simulink model "CONTROL_SYSTEM_V2"  (R2024a)
settings: Solver=ode1  StartTime=0.0  StopTime=inf  FixedStep=0.01  RelTol=1e-5
values from neighbouring files (symbols this model uses):
  B_aet = 0.1503    [ESP32_CONTROL_SYSTEM_VAR_V2.m]
  Beta1 = 3*Omega_o    (= 150)    [ESP32_CONTROL_SYSTEM_VAR_V2.m]
  Beta2 = 3*(Omega_o^2)    (= 7500)    [ESP32_CONTROL_SYSTEM_VAR_V2.m]
  Beta3 = (Omega_o^3)    (= 125000)    [ESP32_CONTROL_SYSTEM_VAR_V2.m]
  Desire_Max = 255    [ESP32_CONTROL_SYSTEM_VAR_V2.m]
  Desire_Min = 0    [ESP32_CONTROL_SYSTEM_VAR_V2.m]
  Direction_Pin = 1    [ESP32_CONTROL_SYSTEM_VAR_V2.m]
  EN_Pin = 0    [ESP32_CONTROL_SYSTEM_VAR_V2.m]
  F_so = 0.089    [ESP32_CONTROL_SYSTEM_VAR_V2.m]
  J_aet = 0.0035    [ESP32_CONTROL_SYSTEM_VAR_V2.m]
  K_sp = 0.038586    [ESP32_CONTROL_SYSTEM_VAR_V2.m]
  Kd = 0.42    [ESP32_CONTROL_SYSTEM_VAR_V2.m]
  Ki = 2    [ESP32_CONTROL_SYSTEM_VAR_V2.m]
  Kp = 3    [ESP32_CONTROL_SYSTEM_VAR_V2.m]
  omga_c = 2    [ESP32_CONTROL_SYSTEM_VAR_V2.m]
  roa = 0.24    [ESP32_CONTROL_SYSTEM_VAR_V2.m]
  theta_o = 12    [ESP32_CONTROL_SYSTEM_VAR_V2.m]
  Toa_ho = 0.3193    [ESP32_CONTROL_SYSTEM_VAR_V2.m]
undefined symbols (not defined in the file or in its folder): Kn, sigbuilder_block
libraries: arduinolib x29, simulink_extras x12, slpidlib x3, spsOnDelayLib x2, simulink x2, slctrl_autotuning x2
(part 3 of 3)

== system CONTROL_SYSTEM_V2/Subsystem2/TB_Feedbakc Range Conversion1 ==
  Control Output : Inport
  TB_maxVal : Inport  Port=2
  TB_minVal : Inport  Port=3
  Add2 : Sum  Inputs=+-
  Add3 : Sum  Inputs=+-
  Constant : Constant
  Constant1 : Constant  Value=0
  Display1 : Display
  Display3 : Display
  Divide1 : Product  Inputs=*/
  Product1 : Product
  Subtract : Sum  Inputs=+-
  Sum : Sum
  0 - 100 Output1 : Outport
  wires:
  Subtract/1 -> Product1/2
  Sum/1 -> 0 - 100 Output1/1
  Product1/1 -> Sum/2
  Constant/1 -> Add2/1
  Add2/1 -> Display1/1, Divide1/1
  Constant1/1 -> Add2/2, Sum/1
  TB_maxVal/1 -> Add3/1
  Add3/1 -> Divide1/2, Display3/1
  Divide1/1 -> Product1/1
  Control Output/1 -> Subtract/1
  TB_minVal/1 -> Subtract/2, Add3/2

== system CONTROL_SYSTEM_V2/Subsystem6/FP_Input Range Conversion2 ==
  Control Output : Inport
  FP_maxVal : Inport  Port=2
  FP_minVal : Inport  Port=3
  Add2 : Sum  Inputs=+-
  Add3 : Sum  Inputs=+-
  Desire Max Value : Constant  Value=Desire_Max
  Desire Min Value : Constant  Value=Desire_Min
  Display1 : Display
  Display3 : Display
  Divide1 : Product  Inputs=*/
  Product1 : Product
  Subtract : Sum  Inputs=+-
  Sum : Sum
  0 - 255 Output : Outport
  wires:
  Control Output/1 -> Subtract/1
  FP_maxVal/1 -> Add3/1
  Add3/1 -> Divide1/2, Display3/1
  FP_minVal/1 -> Subtract/2, Add3/2
  Desire Min Value/1 -> Add2/2, Sum/1
  Subtract/1 -> Product1/2
  Desire Max Value/1 -> Add2/1
  Add2/1 -> Display1/1, Divide1/1
  Divide1/1 -> Product1/1
  Product1/1 -> Sum/2
  Sum/1 -> 0 - 255 Output/1

== system CONTROL_SYSTEM_V2/Subsystem6/H-Bridge Setting2 ==
  1 - 100 : Inport
  Digital Output : arduinolib/Digital Output  pinNumber=0  Direction=output  blockPlatform=arduino
  Digital Output1 : arduinolib/Digital Output  pinNumber=16  Direction=output  blockPlatform=arduino
  Direction Pin : Constant  Value=Direction_Pin
  Display3 : Display
  Display4 : Display
  Enable Pin : Constant  Value=EN_Pin
  PWM : arduinolib/PWM  pinNumber=4  frequencyType=Specify  desiredFrequency=19000  achievableFrequency=19000
  wires:
  Enable Pin/1 -> Display4/1, Digital Output/1
  1 - 100/1 -> PWM/1
  Direction Pin/1 -> Display3/1, Digital Output1/1

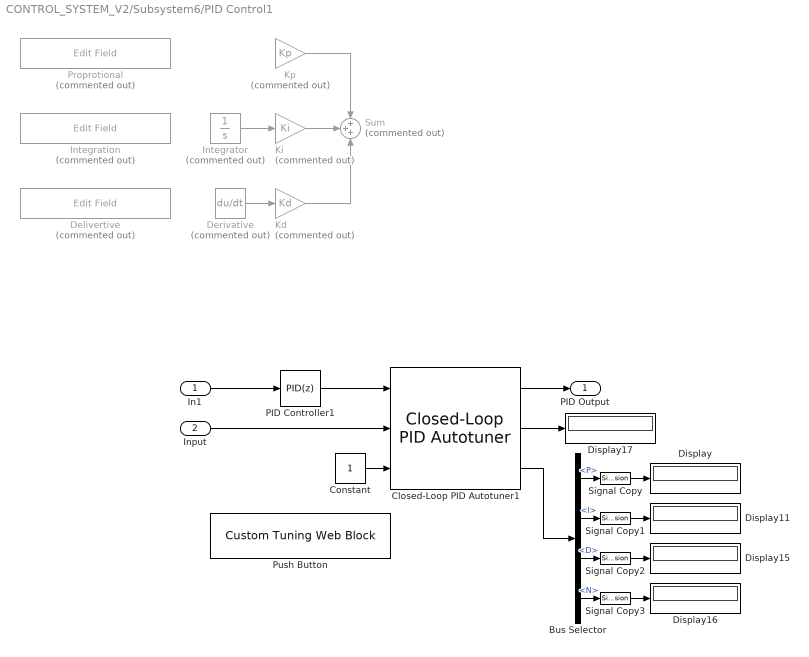
== system CONTROL_SYSTEM_V2/Subsystem6/PID Control1 ==
  In1 : Inport
  Input : Inport  Port=2
  Bus Selector : BusSelector  OutputSignals=P,I,D,N
  Closed-Loop PID Autotuner1 : slctrl_autotuning/Closed-Loop PID Autotuner  PIDType=PI  PIDForm=Parallel  TimeDomain=discrete-time  DiscreteTs=0.1  TuningTs=0.2  UseTuningTs=off  IntegratorFormula=Forward Euler  FilterFormula=Forward Euler  ContinuousTs=0.02  Bandwidth=1  UseExternalWC=off  TargetPM=60  UseExternalPM=off  UseExternalAchievedPM=off  ExperimentMode=Superposition  PlantType=Stable  PlantSign=Positive  AmpSine=1  UseExternalAmpSine=off  UseExternalFRD=off  UseExternalU0=off  UseCompanion=off  NotDeployTuningModule=off  UsePLCCoder=off  OutputMode=control action + perturbation  BlockDataType=double  UseConnectedPID=on  blockpath=[]  tunedP=0  tunedI=0  tunedD=0  tunedN=100  tunedPM=0  EstimationWindowSize=3  UseExternalTuningParams=off  SingleMultiRateVariant=SingleSamplingRate  NumEstimationPeriods=4  NumSettlingPeriods=2  NumOfPRBSPeriod=1  PRBSSignalOrder=12  ExperimentModeVariant=VariantSuperimposed  OutputChoice=VariantCandD
      settings: LibrarySourceBlock=slctrlblks/Autotuning/Closed-Loop PID Autotuner
  Constant : Constant
  Delivertive : EditField  Commented=on  LabelPosition=Hide  ShowInitialText=on  Alignment=Center
  Derivative : Derivative  Commented=on
  Display{,11,15..17} (5 alike) : Display
  Integration : EditField  Commented=on  LabelPosition=Hide  ShowInitialText=on  Alignment=Center
  Integrator : Integrator  Commented=on
  Kd : Gain  Commented=on  Gain=Kd
  Ki : Gain  Commented=on  Gain=Ki
  Kp : Gain  Commented=on  Gain=Kp
  PID Controller1 : slpidlib/PID Controller  Controller=PID  Form=Parallel  TimeDomain=Discrete-time  UseExternalTs=off  SampleTime=-1  IntegratorMethod=Forward Euler  FilterMethod=Forward Euler  ControllerParametersSource=internal  P=1  I=1  UseKiTs=off  D=0  UseExternalDerivativeSource=off  N=100  UseFilter=on  TunerSelectOption=Transfer Function Based (PID Tuner App)  InitialConditionSource=internal  InitialConditionForIntegrator=0  InitialConditionForFilter=0  DifferentiatorICPrevScaledInput=0  ExternalReset=none  TrackingMode=off  Kt=1  LimitOutput=off  SatLimitsSource=internal  UpperSaturationLimit=inf  LowerSaturationLimit=-inf  LinearizeAsGain=on  AntiWindupMode=none  Kb=1  LimitIntegrator=off  UpperIntegratorSaturationLimit=inf  LowerIntegratorSaturationLimit=-inf  POutMin=[]  POutMax=[]  IOutMin=[]  IOutMax=[]  DOutMin=[]  DOutMax=[]  NOutMin=[]  NOutMax=[]  SumOutMin=[]  SumOutMax=[]  SaturationOutMin=[]  SaturationOutMax=[]  PParamMin=[]  PParamMax=[]  IParamMin=[]  IParamMax=[]  DParamMin=[]  DParamMax=[]  NParamMin=[]  NParamMax=[]  KbParamMin=[]  KbParamMax=[]  KtParamMin=[]  KtParamMax=[]  KbOutMin=[]  KbOutMax=[]  KtOutMin=[]  KtOutMax=[]  IntegratorOutMin=[]  IntegratorOutMax=[]  FilterOutMin=[]  FilterOutMax=[]  SumI1OutMin=[]  SumI1OutMax=[]  SumI2OutMin=[]  SumI2OutMax=[]  SumI3OutMin=[]  SumI3OutMax=[]  SumI4OutMin=[]  SumI4OutMax=[]  SumDOutMin=[]  SumDOutMax=[]  DifferentiatorOutMin=[]  DifferentiatorOutMax=[]  FilterDiffOutCoefMin=[]  FilterDiffOutCoefMax=[]  ReciprocalOutMin=[]  ReciprocalOutMax=[]  SumDenOutMin=[]  SumDenOutMax=[]  SumNumOutMin=[]  SumNumOutMax=[]  DivideOutMin=[]  DivideOutMax=[]  UdiffTsProdOutMin=[]  UdiffTsProdOutMax=[]  NTsProdOutMin=[]  NTsProdOutMax=[]  UintegralTsProdOutMin=[]  UintegralTsProdOutMax=[]  UngainTsProdOutMin=[]  UngainTsProdOutMax=[]  ClampingZeroOutDataTypeStr=Inherit: Inherit via back propagation  ClampingZeroOutMin=[]  ClampingZeroOutMax=[]  FilterDenConstantOutDataTypeStr=Inherit: Inherit via back propagation  FilterDenConstantOutMin=[]  FilterDenConstantOutMax=[]  PCopyOutDataTypeStr=Inherit: Inherit via back propagation  PCopyOutMin=[]  PCopyOutMax=[]  NCopyOutDataTypeStr=Inherit: Inherit via back propagation  NCopyOutMin=[]  NCopyOutMax=[]  IntegratorContinuousStateAttributes=''  IntegratorStateMustResolveToSignalObject=off  IntegratorRTWStateStorageClass=Auto  FilterContinuousStateAttributes=''  FilterStateMustResolveToSignalObject=off  FilterRTWStateStorageClass=Auto  ParallelPVariant=InternalParameters  IdealPVariant=Disabled  IVariant=InternalParameters  DVariant=InternalParameters  IntegratorVariant=Discrete  SatVariant=Disabled  AWVariant=Passthrough  PCopyVariant=Disabled  TRVariant=Disabled  FdbkBlocksVariant=Forward  IdealPFdbkVariant=Disabled  SatFdbkVariant=Disabled  DerivativeFilterVariant=ForwardEulerFilter  NVariant=InternalParameters  NCopyVariant=Disabled  FilterICVariant=InternalICsFilter  IntegratorICVariant=InternalICs  ExternalResetVariant=Disabled  TRSumVariant=Passthrough  SumFdbkVariant=Disabled  SumVariant=Sum_PID  TsampFilterVariant=InternalTs  TsampNgainVariant=Passthrough  TsampIntegralVariant=Disabled_SignalSpec  ExternalSaturationOutDataTypeStr=Inherit: Same as second input  DerivativeSourceVariant=ErrorSignal
  Proprotional : EditField  Commented=on  LabelPosition=Hide  ShowInitialText=on  Alignment=Center
  Push Button : CustomTuningWebBlock  LabelPosition=Hide  ShowInitialText=on  Configuration="{\"components\":[{\"name\":\"BackgroundImageComponent\",\"settings\":{\"image\":{\"size\":[0,0],\"src\":\"default\",\"srcOrientation\":\"horizontal\"},\"position\":[0,0,1,1],\"scaleMode\":\"0\"}},{\"name\":\"ButtonStateComponent\",\"settings\":{\"buttonType\":\"latch\",\"clickFcn\":\"\",\"image\":{\"size\":[180,45],\"srcOrientation\":\"Right\"},\"latched\":true,\"offValue\":0,\"onValue\":\"1\",\"position\":[0,0,1,1],\"pressDelay\":\"500\",\"pressFcn\":\"\",\"repeatInterval\":\"0\",\"states\":[{\"horizontalAlignment\":\"center\",\"image\":{\"position\":[0.04444444444444445,0.005555555555555536,0.9888888888888889,0.9111111111111111],\"size\":[0.9888888888888889,0.9111111111111111],\"src\":\"data:image\\/svg+xml;base64,PHN2ZyB4bWxucz0iaHR0cDovL3d3dy53My5vcmcvMjAwMC9zdmciIHhtbG5zOnhsaW5rPSJodHRwOi8vd3d3LnczLm9yZy8xOTk5L3hsaW5rIiB2aWV3Qm94PSIwIDAgMTc3LjI1IDQwLjg4Ij48ZGVmcz48c3R5bGU+LmNscy0xe2ZpbGw6dXJsKCNyYWRpYWwtZ3JhZGllbnQpO30uY2xzLTJ7ZmlsbDp1cmwoI2xpbmVhci1ncmFkaWVudCk7fS5jbHMtM3tmaWxsOnVybCgjbGluZWFyLWdyYWRpZW50LTIpO308L3N0eWxlPjxyYWRpYWxHcmFkaWVudCBpZD0icmFkaWFsLWdyYWRpZW50IiBjeD0iOTAuMDkiIGN5PSIyMi42NiIgcj0i ...(+2212 chars)\",\"srcOrientation\":\"Right\"},\"label\":{\"color\":[1,1,0.78,1],\"icon\":{\"size\":[0.1,0.375],\"src\":\"data:image\\/svg+xml;base64,PHN2ZyBpZD0iT2ZmIiB4bWxucz0iaHR0cDovL3d3dy53My5vcmcvMjAwMC9zdmciIHhtbG5zOnhsaW5rPSJodHRwOi8vd3d3LnczLm9yZy8xOTk5L3hsaW5rIiB2aWV3Qm94PSIwIDAgNTAgNTAiPjxkZWZzPjxzdHlsZT4uY2xzLTF7ZmlsbDojN2Y4MDgwO3N0cm9rZTojMjcyNjI2O3N0cm9rZS1taXRlcmxpbWl0OjEwO3N0cm9rZS13aWR0aDozcHg7fS5jbHMtMntmaWxsOnVybCgjbGluZWFyLWdyYWRpZW50KTt9PC9zdHlsZT48bGluZWFyR3JhZGllbnQgaWQ9ImxpbmVhci1ncmFkaWVudCIgeDE9IjI1IiB5MT0iOSIgeDI9IjI1IiB5Mj0iMzciIGdyYWRpZW50VW5pdHM9InVzZXJTcGFjZU9uVXNlIj48c3RvcCBvZmZzZXQ9IjAiIHN0b3AtY29sb3I9IiNmZmYiIHN0b3Atb3BhY2l0eT0iMC43NSIvPjxzdG9wIG9mZnNldD0iMSIgc3RvcC1jb2xvcj0iI2ZmZiIgc3RvcC1vcGFjaXR5PSIwIi8+PC9saW5lYXJHcmFkaWVudD48L2RlZnM+PGNpcmNsZSBjbGFzcz0iY2xzLTEiIGN4PSIyNSIgY3k9IjI1IiByPSIyMCIvPjxjaXJjbGUgY2xhc3M9ImNscy0yIiBjeD0iMjUiIGN5PSIyMyIgcj0iMTQiLz48L3N2Zz4=\",\"srcOrientation\":\"Right\"},\"iconPlacement\":\"left\",\"opacity\":1,\"show\":true,\"text\":{\"content\":\"Button\",\"font\":\"Helvetica\",\"fontSize\":14}},\"labelOffset\":[0,0],\"verticalAlignment\":\"middle\"},{\"horizontalAlignment\":\"center\",\"image\":{\"position\":[0.04444444444444445,0.005555555555555536,0.9888888888888889,0.9111111111111111],\"size\":[0.9888888888888889,0.9111111111111111],\"src\":\"data:image\\/svg+xml;base64,PHN2ZyB4bWxucz0iaHR0cDovL3d3dy53My5vcmcvMjAwMC9zdmciIHhtbG5zOnhsaW5rPSJodHRwOi8vd3d3LnczLm9yZy8xOTk5L3hsaW5rIiB2aWV3Qm94PSIwIDAgMTc3LjI1IDQwLjg4Ij48ZGVmcz48c3R5bGU+LmNscy0xe2ZpbGw6dXJsKCNyYWRpYWwtZ3JhZGllbnQpO30uY2xzLTJ7ZmlsbDp1cmwoI2xpbmVhci1ncmFkaWVudCk7fS5jbHMtM3tmaWxsOnVybCgjbGluZWFyLWdyYWRpZW50LTIpO308L3N0eWxlPjxyYWRpYWxHcmFkaWVudCBpZD0icmFkaWFsLWdyYWRpZW50IiBjeD0iOTAuMDkiIGN5PSIyMi42NiIgcj0i ...(+2216 chars)\",\"srcOrientation\":\"Right\"},\"label\":{\"color\":[1,1,0.78,1],\"icon\":{\"size\":[0.1,0.375],\"src\":\"data:image\\/svg+xml;base64,PHN2ZyB4bWxucz0iaHR0cDovL3d3dy53My5vcmcvMjAwMC9zdmciIHhtbG5zOnhsaW5rPSJodHRwOi8vd3d3LnczLm9yZy8xOTk5L3hsaW5rIiB2aWV3Qm94PSIwIDAgNTAgNTAiPjxkZWZzPjxzdHlsZT4uY2xzLTF7ZmlsbDojNmFiZDQ1O3N0cm9rZTojMjcyNjI2O3N0cm9rZS1taXRlcmxpbWl0OjEwO3N0cm9rZS13aWR0aDozcHg7fS5jbHMtMntmaWxsOnVybCgjbGluZWFyLWdyYWRpZW50KTt9PC9zdHlsZT48bGluZWFyR3JhZGllbnQgaWQ9ImxpbmVhci1ncmFkaWVudCIgeDE9IjI1IiB5MT0iOSIgeDI9IjI1IiB5Mj0iMzciIGdyYWRpZW50VW5pdHM9InVzZXJTcGFjZU9uVXNlIj48c3RvcCBvZmZzZXQ9IjAiIHN0b3AtY29sb3I9IiNmZmYiIHN0b3Atb3BhY2l0eT0iMC43NSIvPjxzdG9wIG9mZnNldD0iMSIgc3RvcC1jb2xvcj0iI2ZmZiIgc3RvcC1vcGFjaXR5PSIwIi8+PC9saW5lYXJHcmFkaWVudD48L2RlZnM+PGcgaWQ9Ik9uIj48Y2lyY2xlIGNsYXNzPSJjbHMtMSIgY3g9IjI1IiBjeT0iMjUiIHI9IjIwIi8+PGNpcmNsZSBjbGFzcz0iY2xzLTIiIGN4PSIyNSIgY3k9IjIzIiByPSIxNCIvPjwvZz48L3N2Zz4=\",\"srcOrientation\":\"Right\"},\"iconPlacement\":\"left\",\"opacity\":1,\"show\":true,\"text\":{\"content\":\"Button\",\"font\":\"Helvetica\",\"fontSize\":14}},\"labelOffset\":[0.025,0],\"verticalAlignment\":\"middle\"},{\"horizontalAlignment\":\"center\",\"image\":{\"position\":[0.04444444444444445,0.005555555555555536,0.9888888888888889,0.9111111111111111],\"size\":[0.9888888888888889,0.9111111111111111],\"src\":\"data:image\\/svg+xml;base64,PHN2ZyB4bWxucz0iaHR0cDovL3d3dy53My5vcmcvMjAwMC9zdmciIHhtbG5zOnhsaW5rPSJodHRwOi8vd3d3LnczLm9yZy8xOTk5L3hsaW5rIiB2aWV3Qm94PSIwIDAgMTc3LjI1IDQwLjg4Ij48ZGVmcz48c3R5bGU+LmNscy0xe2ZpbGw6dXJsKCNyYWRpYWwtZ3JhZGllbnQpO30uY2xzLTJ7ZmlsbDp1cmwoI2xpbmVhci1ncmFkaWVudCk7fS5jbHMtM3tmaWxsOnVybCgjbGluZWFyLWdyYWRpZW50LTIpO308L3N0eWxlPjxyYWRpYWxHcmFkaWVudCBpZD0icmFkaWFsLWdyYWRpZW50IiBjeD0iOTAuMDkiIGN5PSIyMi42NiIgcj0i ...(+2212 chars)\",\"srcOrientation\":\"Right\"},\"label\":{\"color\":[1,1,0.78,1],\"icon\":{\"size\":[0.1,0.375],\"src\":\"data:image\\/svg+xml;base64,PHN2ZyB4bWxucz0iaHR0cDovL3d3dy53My5vcmcvMjAwMC9zdmciIHhtbG5zOnhsaW5rPSJodHRwOi8vd3d3LnczLm9yZy8xOTk5L3hsaW5rIiB2aWV3Qm94PSIwIDAgNTAgNTAiPjxkZWZzPjxzdHlsZT4uY2xzLTF7ZmlsbDojNmFiZDQ1O3N0cm9rZTojMjcyNjI2O3N0cm9rZS1taXRlcmxpbWl0OjEwO3N0cm9rZS13aWR0aDozcHg7fS5jbHMtMntmaWxsOnVybCgjbGluZWFyLWdyYWRpZW50KTt9PC9zdHlsZT48bGluZWFyR3JhZGllbnQgaWQ9ImxpbmVhci1ncmFkaWVudCIgeDE9IjI1IiB5MT0iOSIgeDI9IjI1IiB5Mj0iMzciIGdyYWRpZW50VW5pdHM9InVzZXJTcGFjZU9uVXNlIj48c3RvcCBvZmZzZXQ9IjAiIHN0b3AtY29sb3I9IiNmZmYiIHN0b3Atb3BhY2l0eT0iMC43NSIvPjxzdG9wIG9mZnNldD0iMSIgc3RvcC1jb2xvcj0iI2ZmZiIgc3RvcC1vcGFjaXR5PSIwIi8+PC9saW5lYXJHcmFkaWVudD48L2RlZnM+PGcgaWQ9Ik9uIj48Y2lyY2xlIGNsYXNzPSJjbHMtMSIgY3g9IjI1IiBjeT0iMjUiIHI9IjIwIi8+PGNpcmNsZSBjbGFzcz0iY2xzLTIiIGN4PSIyNSIgY3k9IjIzIiByPSIxNCIvPjwvZz48L3N2Zz4=\",\"srcOrientation\":\"Right\"},\"iconPlacement\":\"left\",\"opacity\":1,\"show\":true,\"text\":{\"content\":\"Button\",\"font\":\"Helvetica\",\"fontSize\":14}},\"labelOffset\":[0,0],\"verticalAlignment\":\"middle\"},{\"horizontalAlignment\":\"center\",\"image\":{\"position\":[0.04444444444444445,0.005555555555555536,0.9888888888888889,0.9111111111111111],\"size\":[0.9888888888888889,0.9111111111111111],\"src\":\"data:image\\/svg+xml;base64,PHN2ZyB4bWxucz0iaHR0cDovL3d3dy53My5vcmcvMjAwMC9zdmciIHhtbG5zOnhsaW5rPSJodHRwOi8vd3d3LnczLm9yZy8xOTk5L3hsaW5rIiB2aWV3Qm94PSIwIDAgMTc3LjI1IDQwLjg4Ij48ZGVmcz48c3R5bGU+LmNscy0xe2ZpbGw6dXJsKCNyYWRpYWwtZ3JhZGllbnQpO30uY2xzLTJ7ZmlsbDp1cmwoI2xpbmVhci1ncmFkaWVudCk7fS5jbHMtM3tmaWxsOnVybCgjbGluZWFyLWdyYWRpZW50LTIpO308L3N0eWxlPjxyYWRpYWxHcmFkaWVudCBpZD0icmFkaWFsLWdyYWRpZW50IiBjeD0iOTAuMDkiIGN5PSIyMi42NiIgcj0i ...(+2216 chars)\",\"srcOrientation\":\"Right\"},\"label\":{\"color\":[1,1,0.78,1],\"icon\":{\"size\":[0.1,0.375],\"src\":\"data:image\\/svg+xml;base64,PHN2ZyBpZD0iT2ZmIiB4bWxucz0iaHR0cDovL3d3dy53My5vcmcvMjAwMC9zdmciIHhtbG5zOnhsaW5rPSJodHRwOi8vd3d3LnczLm9yZy8xOTk5L3hsaW5rIiB2aWV3Qm94PSIwIDAgNTAgNTAiPjxkZWZzPjxzdHlsZT4uY2xzLTF7ZmlsbDojN2Y4MDgwO3N0cm9rZTojMjcyNjI2O3N0cm9rZS1taXRlcmxpbWl0OjEwO3N0cm9rZS13aWR0aDozcHg7fS5jbHMtMntmaWxsOnVybCgjbGluZWFyLWdyYWRpZW50KTt9PC9zdHlsZT48bGluZWFyR3JhZGllbnQgaWQ9ImxpbmVhci1ncmFkaWVudCIgeDE9IjI1IiB5MT0iOSIgeDI9IjI1IiB5Mj0iMzciIGdyYWRpZW50VW5pdHM9InVzZXJTcGFjZU9uVXNlIj48c3RvcCBvZmZzZXQ9IjAiIHN0b3AtY29sb3I9IiNmZmYiIHN0b3Atb3BhY2l0eT0iMC43NSIvPjxzdG9wIG9mZnNldD0iMSIgc3RvcC1jb2xvcj0iI2ZmZiIgc3RvcC1vcGFjaXR5PSIwIi8+PC9saW5lYXJHcmFkaWVudD48L2RlZnM+PGNpcmNsZSBjbGFzcz0iY2xzLTEiIGN4PSIyNSIgY3k9IjI1IiByPSIyMCIvPjxjaXJjbGUgY2xhc3M9ImNscy0yIiBjeD0iMjUiIGN5PSIyMyIgcj0iMTQiLz48L3N2Zz4=\",\"srcOrientation\":\"Right\"},\"iconPlacement\":\"left\",\"opacity\":1,\"show\":true,\"text\":{\"content\":\"Button\",\"font\":\"Helvetica\",\"fontSize\":14}},\"labelOffset\":[0.025,0],\"verticalAlignment\":\"middle\"}]}},{\"name\":\"ForegroundImageComponent\",\"settings\":{\"image\":{\"size\":[0,0],\"src\":\"default\",\"srcOrientation\":\"horizontal\"},\"isForeground\":1,\"position\":[0,0,1,1],\"scaleMode\":\"0\"}}],\"settings\":{\"BindingType\":\"param\",\"aspectRatio\":3.7777777777777777,\"backgroundColor\":[0,0,0,\"1\"],\"backgroundOffset\":0,\"backgroundOpacity\":1,\"fixedAspectRatio\":\"on\",\"foregroundColor\":[252,252,196],\"showBackgroundColor\":false,\"variant\":\"push\",\"version\":\"R2023a\"},\"type\":\"Button\"}"
  Signal Copy{,1..3} (4 alike) : SignalConversion  OverrideOpt=off
  Sum : Sum  Commented=on  Inputs=+++
  PID Output : Outport
  wires:
  Integrator/1 -> Ki/1
  Kp/1 -> Sum/1
  Ki/1 -> Sum/2
  Derivative/1 -> Kd/1
  Kd/1 -> Sum/3
  PID Controller1/1 -> Closed-Loop PID Autotuner1/1
  Signal Copy3/1 -> Display16/1
  Bus Selector/1 -> Signal Copy/1  "<P>"
  Bus Selector/2 -> Signal Copy1/1  "<I>"
  Signal Copy1/1 -> Display11/1
  Bus Selector/4 -> Signal Copy3/1  "<N>"
  Signal Copy2/1 -> Display15/1
  Signal Copy/1 -> Display/1
  Closed-Loop PID Autotuner1/3 -> Bus Selector/1
  Bus Selector/3 -> Signal Copy2/1  "<D>"
  Input/1 -> Closed-Loop PID Autotuner1/2
  Constant/1 -> Closed-Loop PID Autotuner1/3
  Closed-Loop PID Autotuner1/1 -> PID Output/1
  In1/1 -> PID Controller1/1
  Closed-Loop PID Autotuner1/2 -> Display17/1

== system CONTROL_SYSTEM_V2/Subsystem6/TB_Feedbakc Range Conversion1 ==
  Control Output : Inport
  TB_maxVal : Inport  Port=2
  TB_minVal : Inport  Port=3
  FP_maxVal : Inport  Port=4
  FP_minVal : Inport  Port=5
  Add2 : Sum  Inputs=+-
  Add3 : Sum  Inputs=+-
  Display1 : Display
  Display3 : Display
  Divide1 : Product  Inputs=*/
  Product1 : Product
  Subtract : Sum  Inputs=+-
  Sum : Sum
  0 - 100 Output1 : Outport
  wires:
  Subtract/1 -> Product1/2
  Sum/1 -> 0 - 100 Output1/1
  Product1/1 -> Sum/2
  FP_maxVal/1 -> Add2/1
  Add2/1 -> Display1/1, Divide1/1
  FP_minVal/1 -> Add2/2, Sum/1
  TB_maxVal/1 -> Add3/1
  Add3/1 -> Divide1/2, Display3/1
  Divide1/1 -> Product1/1
  Control Output/1 -> Subtract/1
  TB_minVal/1 -> Subtract/2, Add3/2

== matlab function CONTROL_SYSTEM_V2/Foot Pedal Calibration1 ==
  settings: updateMethod=DISCRETE
  data: PedalRange input; FP_maxVal output; FP_minVal output
function [FP_maxVal, FP_minVal] = FootPadel_Range(PedalRange)
    persistent maxSet minSet;
    if isempty(maxSet)  
        maxSet = -1;
    end
    if isempty(minSet)
        minSet = 5; 
    end
    if PedalRange > maxSet
        maxSet = PedalRange;
    end
    if PedalRange < minSet
        minSet = PedalRange;
    end
    FP_maxVal = maxSet;
    FP_minVal = minSet;
end

== matlab function CONTROL_SYSTEM_V2/Subsystem1/MATLAB Function ==
  data: Pedal_Val input; Desire_Val output
function Desire_Val = fcn(Pedal_Val)

persistent Previous_Val Set_Val
if isempty(Set_Val)
    Set_Val = 0;
end
if isempty(Previous_Val)
    Previous_Val = 0;
else
    Set_Val = abs(Previous_Val - Pedal_Val);
    Previous_Val = Pedal_Val;
end
Desire_Val = abs(Set_Val);
end

== matlab function CONTROL_SYSTEM_V2/Subsystem2/Throttle Body Callibration1 ==
  settings: updateMethod=DISCRETE
  data: TBRange input; TB_maxVal output; TB_minVal output
function [TB_maxVal, TB_minVal] = ThrottleBody_Range(TBRange)
    persistent TB_maxSet TB_minSet;
    if isempty(TB_maxSet)
        TB_maxSet = 0;
    end
    if isempty(TB_minSet)
        TB_minSet = 5; 
    end
    if TBRange > TB_maxSet
        TB_maxSet = TBRange;
    end
    if TBRange < TB_minSet
        TB_minSet = TBRange;
    end
    TB_maxVal = TB_maxSet;
    TB_minVal = TB_minSet;
end

== matlab function CONTROL_SYSTEM_V2/Subsystem6/Pedal Calibration1 ==
  settings: updateMethod=DISCRETE
  data: PedalRange input; FP_maxVal output; FP_minVal output
function [FP_maxVal, FP_minVal] = FootPadel_Range(PedalRange)
    persistent maxSet minSet;
    if isempty(maxSet)
        maxSet = -1;
    end
    if isempty(minSet)
        minSet = 5; 
    end
    if PedalRange > maxSet
        maxSet = PedalRange;
    end
    if PedalRange < minSet
        minSet = PedalRange;
    end
    FP_maxVal = maxSet;
    FP_minVal = minSet;
end

== matlab function CONTROL_SYSTEM_V2/Subsystem4/Pedal Calibration2 ==
  settings: updateMethod=DISCRETE
  data: PedalRange input; FP_maxVal output; FP_minVal output; Calibration_Input input
function [FP_maxVal, FP_minVal] = FootPadel_Range(PedalRange, Calibration_Input)
    persistent maxSet minSet;
    if isempty(maxSet)
        maxSet = 0;
    end
    if isempty(minSet)
        minSet = 5;
    end
    if PedalRange > maxSet
        maxSet = PedalRange;
    end
    if PedalRange < minSet
        minSet = PedalRange;
    end
    FP_maxVal = maxSet;
    FP_minVal = minSet;
    if Calibration_Input == 1
        maxSet = 0;
        minSet = 5;
    end
end

== matlab function CONTROL_SYSTEM_V2/Subsystem6/Throttle Body Callibration2 ==
  settings: updateMethod=DISCRETE
  data: TBRange input; TB_maxVal output; TB_minVal output
function [TB_maxVal, TB_minVal] = ThrottleBody_Range(TBRange)
    persistent TB_maxSet TB_minSet;
    if isempty(TB_maxSet)
        TB_maxSet = 0;
    end
    if isempty(TB_minSet)
        TB_minSet = 5; 
    end
    if TBRange > TB_maxSet
        TB_maxSet = TBRange;
    end
    if TBRange < TB_minSet
        TB_minSet = TBRange;
    end
    TB_maxVal = TB_maxSet;
    TB_minVal = TB_minSet;
end

== matlab function CONTROL_SYSTEM_V2/Subsystem4/Throttle Body Callibration1 ==
  settings: updateMethod=DISCRETE
  data: TBRange input; TB_maxVal output; TB_minVal output; Calibration_Input input
function [TB_maxVal, TB_minVal] = ThrottleBody_Range(TBRange, Calibration_Input)
    persistent TB_maxSet TB_minSet;
    if isempty(TB_maxSet)
        TB_maxSet = 0;
    end
    if isempty(TB_minSet)
        TB_minSet = 5;
    end
    if TBRange > TB_maxSet
        TB_maxSet = TBRange;
    end
    if TBRange < TB_minSet
        TB_minSet = TBRange;
    end
    TB_maxVal = TB_maxSet;
    TB_minVal = TB_minSet;
    if Calibration_Input == 1
        TB_maxSet = 0;
        TB_minSet = 5;
    end
end

== matlab function CONTROL_SYSTEM_V2/Foot Pedal Calibration ==
  settings: updateMethod=DISCRETE
  data: PedalRange input; FP_maxVal output; FP_minVal output
function [FP_maxVal, FP_minVal] = FootPadel_Range(PedalRange)
    % Define a function FootPadel_Range that accepts a pedal position input (PedalRange)
    % and outputs the maximum and minimum values of the pedal position observed so far.
    
    % persistent variables to store maximum and minimum pedal values
    persistent maxSet minSet;
    
    % Initialize maxSet if it hasn't been set yet.
    if isempty(maxSet)
        maxSet = -1;  % Start with a value lower than the minimum possible PedalRange
    end
    
    % Initialize minSet if it hasn't been set yet.
    if isempty(minSet)
        minSet = 5;  % Start with a value higher than the maximum possible PedalRange
    end
    
    % Update maxSet if the current PedalRange is greater than the previous maxSet.
    if PedalRange > maxSet
        maxSet = PedalRange;
    end
    
    % Update minSet if the current PedalRange is less than the previous minSet.
    if PedalRange < minSet
        minSet = PedalRange;
    end
    
    % Assign the maximum and minimum values to the output variables.
    FP_maxVal = maxSet;
    FP_minVal = minSet;
end


% persistent maxSet minSet;: The persistent keyword is used to declare variables that retain their values between function calls. This is crucial for keeping track of the maximum and minimum pedal positions as the function is called multiple times.

% if isempty(maxSet) ... if isempty(minSet): These conditions ensure that the persistent variables are initialized only once, the first time the function is called.

% maxSet = PedalRange; minSet = PedalRange;: The maximum and minimum values are updated whenever a new extreme is found.

% FP_maxVal, FP_minVal: These output variables store the maximum and minimum pedal values, which are returned to the caller.

== matlab function CONTROL_SYSTEM_V2/Throttle Body Callibration ==
  settings: updateMethod=DISCRETE
  data: TB_Range input; TB_maxVal output; TB_minVal output
function [TB_maxVal, TB_minVal] = ThrottleBody_Range(TB_Range)
    % Define a function ThrottleBody_Range that accepts a throttle body position input (TB_Range)
    % and outputs the maximum and minimum values of the throttle position observed so far.
    
    % Persistent variables to store maximum and minimum throttle body values
    persistent TB_maxSet TB_minSet;
    
    % Initialize TB_maxSet if it hasn't been set yet.
    if isempty(TB_maxSet)
        TB_maxSet = -1;  % Start with a value lower than the minimum possible TB_Range
    end
    
    % Initialize TB_minSet if it hasn't been set yet.
    if isempty(TB_minSet)
        TB_minSet = 5;  % Start with a value higher than the maximum possible TB_Range
    end
    
    % Update TB_maxSet if the current TB_Range is greater than the previous TB_maxSet.
    if TB_Range > TB_maxSet
        TB_maxSet = TB_Range;
    end
    
    % Update TB_minSet if the current TB_Range is less than the previous TB_minSet.
    if TB_Range < TB_minSet
        TB_minSet = TB_Range;
    end
    
    % Assign the maximum and minimum values to the output variables.
    TB_maxVal = TB_maxSet;
    TB_minVal = TB_minSet;
end

% persistent TB_maxSet TB_minSet: These persistent variables store the maximum and minimum throttle body positions. They retain their values across multiple calls to the function, allowing the function to keep track of the extremes over time.

% TB_maxSet = -1; TB_minSet = 5: These initial values are set to ensure that the first input will properly update the maximum and minimum values.

% TB_maxVal = TB_maxSet; TB_minVal = TB_minSet: These output variables return the current maximum and minimum throttle body values.

== matlab function CONTROL_SYSTEM_V2/Throttle Body Callibration1 ==
  settings: updateMethod=DISCRETE
  data: TB_Range input; TB_maxVal output; TB_minVal output
function [TB_maxVal, TB_minVal] = ThrottleBody_Range(TB_Range)
    persistent TB_maxSet TB_minSet;
    if isempty(TB_maxSet)
        TB_maxSet = -1;
    end
    if isempty(TB_minSet)
        TB_minSet = 5; 
    end
    if TB_Range > TB_maxSet
        TB_maxSet = TB_Range;
    end
    if TB_Range < TB_minSet
        TB_minSet = TB_Range;
    end
    TB_maxVal = TB_maxSet;
    TB_minVal = TB_minSet;
end
